simulink model "IdentificareBuclaExterna"  (R2023b)
settings: Solver=FixedStepAuto  StartTime=0.0  StopTime=2500  FixedStep=0.01  RelTol=1e-3
values from neighbouring files (symbols this model uses):
  A = 332.5    [CodDatepersonale.m]    (also in CodProiect.m; untitled.m; untitled2.m = [O I; O O]; untitled22.m)
  C = 7.4    [CodDatepersonale.m]    (also in CodProiect.m = 9; untitled.m; untitled22.m = 9)
  k = 0.036    [CodDatepersonale.m]    (also in CodProiect.m = 0.035; untitled.m; untitled22.m = 0.035)
  k1 = 0.624    [CodDatepersonale.m]    (also in CodProiect.m = 0.654; untitled.m = 0.654; untitled22.m)
  k2 = -0.015    [CodDatepersonale.m]    (also in CodProiect.m; untitled.m; untitled22.m)
  k3 = -0.0006    [CodDatepersonale.m]    (also in CodProiect.m; untitled.m; untitled22.m)
  keta = 8*10^(-5)    (= 8e-05)    [CodDatepersonale.m]    (also in CodProiect.m; untitled.m; untitled22.m)
libraries: slpidlib x1
settings Model: Creator=Daniela  LastModifiedBy=Daniela

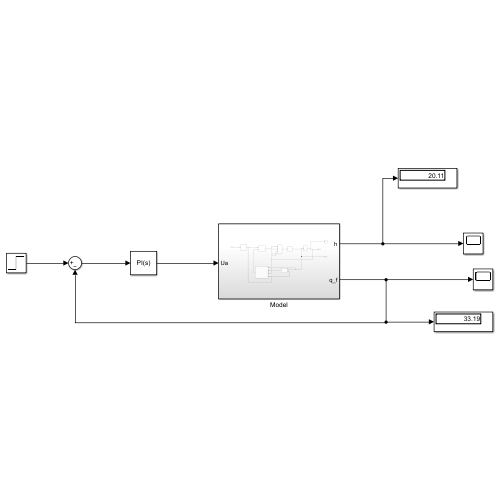
[thumbnail: Simulink's stored preview of the top-level diagram]
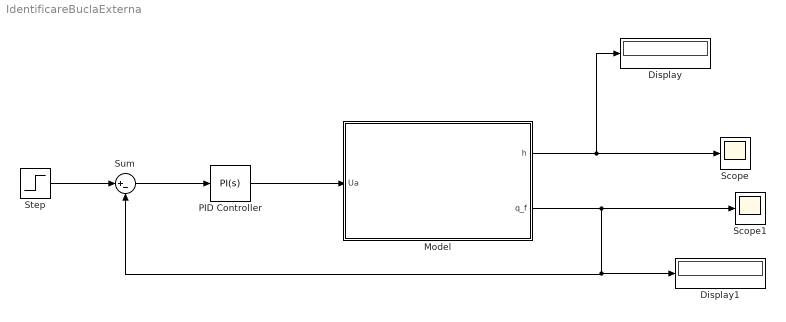
== system IdentificareBuclaExterna ==
  Display : Display
  Display1 : Display
  Model : Subsystem
  PID Controller : slpidlib/PID Controller  Controller=PI  Form=Parallel  TimeDomain=Continuous-time  UseExternalTs=off  SampleTime=-1  IntegratorMethod=Forward Euler  FilterMethod=Forward Euler  ControllerParametersSource=internal  P=0.0698  I=0.0698*1/0.784  UseKiTs=off  D=0  N=100  UseFilter=on  TunerSelectOption=Transfer Function Based (PID Tuner App)  InitialConditionSource=internal  InitialConditionForIntegrator=5.6  InitialConditionForFilter=0  DifferentiatorICPrevScaledInput=0  ExternalReset=none  TrackingMode=off  Kt=1  LimitOutput=off  SatLimitsSource=internal  UpperSaturationLimit=inf  LowerSaturationLimit=-inf  LinearizeAsGain=on  AntiWindupMode=none  Kb=1  LimitIntegrator=off  UpperIntegratorSaturationLimit=inf  LowerIntegratorSaturationLimit=-inf  POutMin=[]  POutMax=[]  IOutMin=[]  IOutMax=[]  DOutMin=[]  DOutMax=[]  NOutMin=[]  NOutMax=[]  SumOutMin=[]  SumOutMax=[]  SaturationOutMin=[]  SaturationOutMax=[]  PParamMin=[]  PParamMax=[]  IParamMin=[]  IParamMax=[]  DParamMin=[]  DParamMax=[]  NParamMin=[]  NParamMax=[]  KbParamMin=[]  KbParamMax=[]  KtParamMin=[]  KtParamMax=[]  KbOutMin=[]  KbOutMax=[]  KtOutMin=[]  KtOutMax=[]  IntegratorOutMin=[]  IntegratorOutMax=[]  FilterOutMin=[]  FilterOutMax=[]  SumI1OutMin=[]  SumI1OutMax=[]  SumI2OutMin=[]  SumI2OutMax=[]  SumI3OutMin=[]  SumI3OutMax=[]  SumI4OutMin=[]  SumI4OutMax=[]  SumDOutMin=[]  SumDOutMax=[]  DifferentiatorOutMin=[]  DifferentiatorOutMax=[]  FilterDiffOutCoefMin=[]  FilterDiffOutCoefMax=[]  ReciprocalOutMin=[]  ReciprocalOutMax=[]  SumDenOutMin=[]  SumDenOutMax=[]  SumNumOutMin=[]  SumNumOutMax=[]  DivideOutMin=[]  DivideOutMax=[]  UdiffTsProdOutMin=[]  UdiffTsProdOutMax=[]  NTsProdOutMin=[]  NTsProdOutMax=[]  UintegralTsProdOutMin=[]  UintegralTsProdOutMax=[]  UngainTsProdOutMin=[]  UngainTsProdOutMax=[]  ClampingZeroOutDataTypeStr=Inherit: Inherit via back propagation  ClampingZeroOutMin=[]  ClampingZeroOutMax=[]  FilterDenConstantOutDataTypeStr=Inherit: Inherit via back propagation  FilterDenConstantOutMin=[]  FilterDenConstantOutMax=[]  PCopyOutDataTypeStr=Inherit: Inherit via back propagation  PCopyOutMin=[]  PCopyOutMax=[]  NCopyOutDataTypeStr=Inherit: Inherit via back propagation  NCopyOutMin=[]  NCopyOutMax=[]  IntegratorContinuousStateAttributes=''  IntegratorStateMustResolveToSignalObject=off  IntegratorRTWStateStorageClass=Auto  FilterContinuousStateAttributes=''  FilterStateMustResolveToSignalObject=off  FilterRTWStateStorageClass=Auto  ParallelPVariant=InternalParameters  IdealPVariant=Disabled  IVariant=InternalParameters  DVariant=Disabled  IntegratorVariant=Continuous  SatVariant=Disabled  AWVariant=Passthrough  PCopyVariant=Disabled  TRVariant=Disabled  FdbkBlocksVariant=Forward  IdealPFdbkVariant=Disabled  SatFdbkVariant=Disabled  DerivativeFilterVariant=Disabled  NVariant=Disabled  NCopyVariant=Disabled_SignalSpec  FilterICVariant=Disabled  IntegratorICVariant=InternalICs  ExternalResetVariant=Disabled  TRSumVariant=Passthrough  SumFdbkVariant=Disabled  SumVariant=Sum_PI  TsampFilterVariant=InternalTs  TsampNgainVariant=Passthrough  TsampIntegralVariant=Disabled_SignalSpec  ExternalSaturationOutDataTypeStr=Inherit: Same as second input
  Scope : Scope
  Scope1 : Scope
  Step : Step  Time=0  Before=30.22  After=33.19  SampleTime=0
  Sum : Sum  Inputs=|+-
  wires:
  PID Controller/1 -> Model/1(Ua)
  Model/1(h) -> Display/1, Scope/1
  Model/2(q_f) -> Sum/2, Display1/1, Scope1/1
  Sum/1 -> PID Controller/1
  Step/1 -> Sum/1

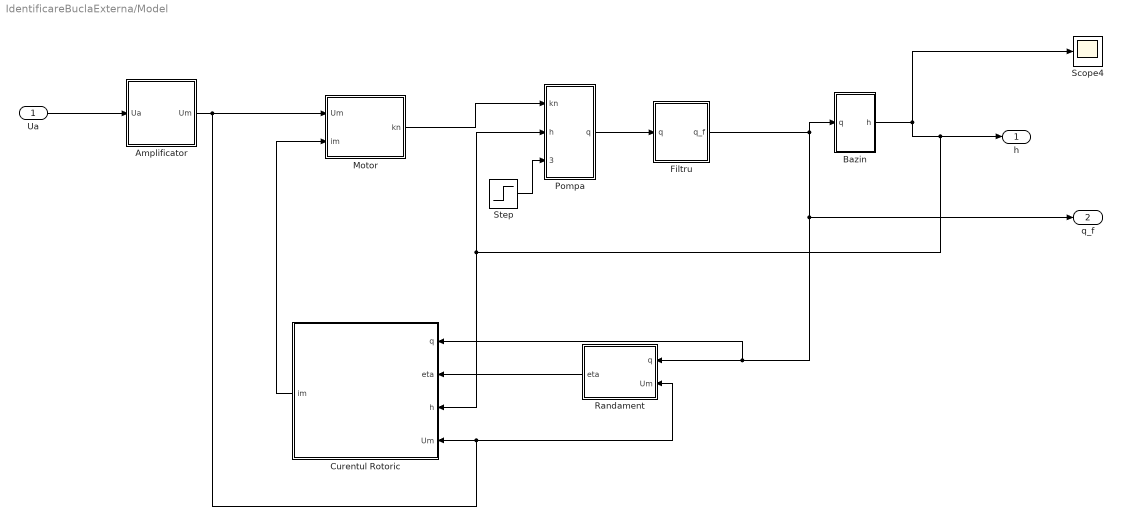
== system IdentificareBuclaExterna/Model ==
  Ua : Inport
  Amplificator : Subsystem
  Bazin : Subsystem
  Curentul Rotoric : Subsystem
  Filtru : Subsystem
  Motor : Subsystem
  Pompa : Subsystem
  Randament : Subsystem
  Scope4 : Scope
  Step : Step  Time=250  After=0.0036  SampleTime=0
  h : Outport
  q_f : Outport  Port=2
  wires:
  Bazin/1(h) -> Scope4/1, h/1, Pompa/2(h), Curentul Rotoric/3(h)
  Randament/1(eta) -> Curentul Rotoric/2(eta)
  Pompa/1(q) -> Filtru/1(q)
  Ua/1 -> Amplificator/1(Ua)
  Step/1 -> Pompa/3(Perturbatie k)
  Motor/1(kn) -> Pompa/1(kn)
  Filtru/1(q_f) -> q_f/1, Randament/1(q), Curentul Rotoric/1(q), Bazin/1(q)
  Curentul Rotoric/1(im) -> Motor/2(im)
  Amplificator/1(Um) -> Motor/1(Um), Randament/2(Um), Curentul Rotoric/4(Um)

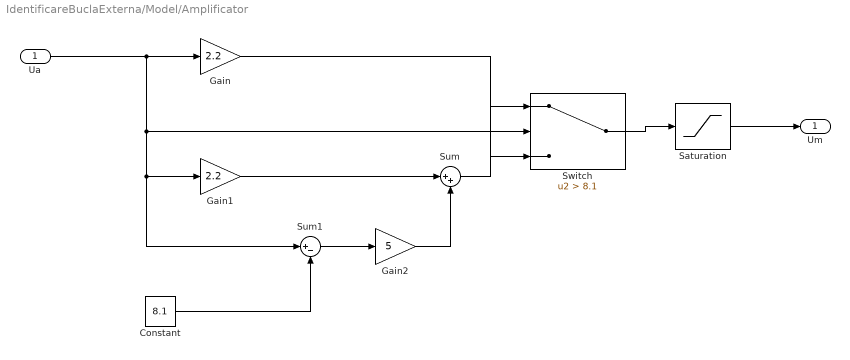
== system IdentificareBuclaExterna/Model/Amplificator ==
  Ua : Inport
  Constant : Constant  Value=8.1
  Gain : Gain  Gain=2.2
  Gain1 : Gain  Gain=2.2
  Gain2 : Gain  Gain=5
  Saturation : Saturate  UpperLimit=22  LowerLimit=0  ZeroCross=off
  Sum : Sum  Inputs=|++
  Sum1 : Sum  Inputs=|+-
  Switch : Switch  Criteria=u2 > Threshold  Threshold=8.1  SaturateOnIntegerOverflow=off  InputSameDT=off
  Um : Outport
  wires:
  Switch/1 -> Saturation/1
  Ua/1 -> Sum1/1, Gain1/1, Switch/2, Gain/1
  Constant/1 -> Sum1/2
  Sum1/1 -> Gain2/1
  Gain/1 -> Switch/3
  Sum/1 -> Switch/1
  Gain1/1 -> Sum/1
  Gain2/1 -> Sum/2
  Saturation/1 -> Um/1

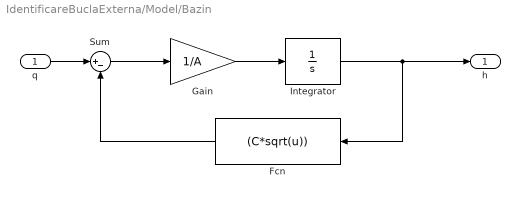
== system IdentificareBuclaExterna/Model/Bazin ==
  q : Inport
  Fcn : Fcn  Expr=(C*sqrt(u))
  Gain : Gain  Gain=1/A
  Integrator : Integrator  InitialCondition=16.53
  Sum : Sum  Inputs=|+-
  h : Outport
  wires:
  q/1 -> Sum/1
  Sum/1 -> Gain/1
  Fcn/1 -> Sum/2
  Gain/1 -> Integrator/1
  Integrator/1 -> h/1, Fcn/1

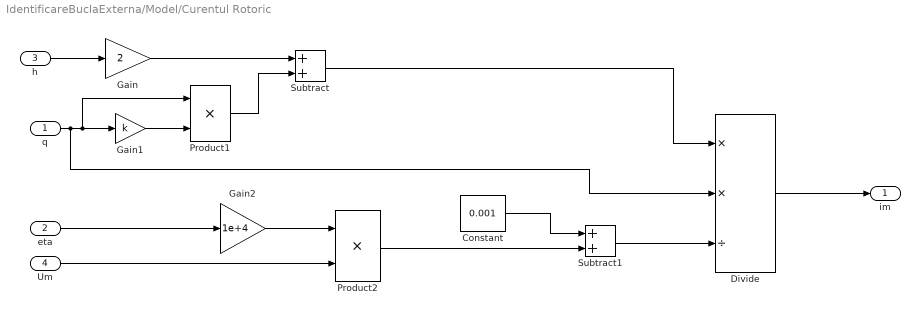
== system IdentificareBuclaExterna/Model/Curentul Rotoric ==
  q : Inport
  eta : Inport  Port=2
  h : Inport  Port=3
  Um : Inport  Port=4
  Constant : Constant  Value=0.001
  Divide : Product  Inputs=**/
  Gain : Gain  Gain=2
  Gain1 : Gain  Gain=k
  Gain2 : Gain  Gain=1e+4
  Product1 : Product
  Product2 : Product
  Subtract : Sum
  Subtract1 : Sum
  im : Outport
  wires:
  Product1/1 -> Subtract/2
  Um/1 -> Product2/2
  q/1 -> Gain1/1, Product1/1, Divide/2
  Subtract/1 -> Divide/1
  Divide/1 -> im/1
  Subtract1/1 -> Divide/3
  Gain2/1 -> Product2/1
  h/1 -> Gain/1
  Gain/1 -> Subtract/1
  Gain1/1 -> Product1/2
  eta/1 -> Gain2/1
  Product2/1 -> Subtract1/2
  Constant/1 -> Subtract1/1

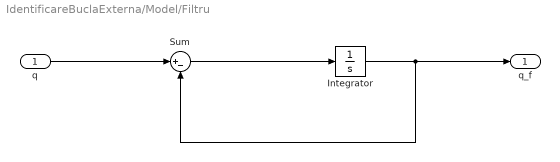
== system IdentificareBuclaExterna/Model/Filtru ==
  q : Inport
  Integrator : Integrator  InitialCondition=30.22
  Sum : Sum  Inputs=|+-
  q_f : Outport
  wires:
  Integrator/1 -> q_f/1, Sum/2
  q/1 -> Sum/1
  Sum/1 -> Integrator/1

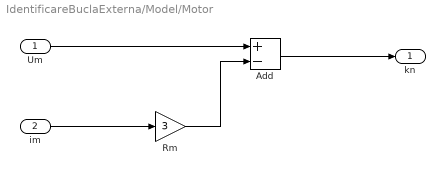
== system IdentificareBuclaExterna/Model/Motor ==
  Um : Inport
  im : Inport  Port=2
  Add : Sum  Inputs=+-
  Rm : Gain  Gain=3
  kn : Outport
  wires:
  im/1 -> Rm/1
  Add/1 -> kn/1
  Um/1 -> Add/1
  Rm/1 -> Add/2

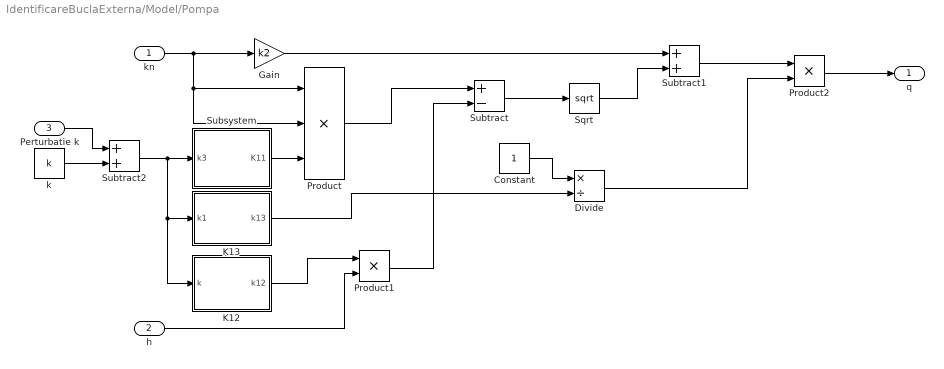
== system IdentificareBuclaExterna/Model/Pompa ==
  kn : Inport
  h : Inport  Port=2
  Perturbatie k : Inport  Port=3
  Constant : Constant
  Divide : Product  Inputs=*/
  Gain : Gain  Gain=k2
  K12 : Subsystem
  K13 : Subsystem
  Product : Product  Inputs=3
  Product1 : Product
  Product2 : Product
  Sqrt : Sqrt
  Subsystem : Subsystem
  Subtract : Sum  Inputs=+-
  Subtract1 : Sum
  Subtract2 : Sum
  k : Constant  Value=k
  q : Outport
  wires:
  K12/1(k12) -> Product1/1
  Product2/1 -> q/1
  Subtract1/1 -> Product2/1
  Product/1 -> Subtract/1
  Subtract/1 -> Sqrt/1
  Divide/1 -> Product2/2
  Product1/1 -> Subtract/2
  Subtract2/1 -> Subsystem/1(k3), K12/1(k), K13/1(k1)
  k/1 -> Subtract2/2
  K13/1(k13) -> Divide/2
  Perturbatie k/1 -> Subtract2/1
  Gain/1 -> Subtract1/1
  Subsystem/1(K11) -> Product/3
  Constant/1 -> Divide/1
  h/1 -> Product1/2
  Sqrt/1 -> Subtract1/2
  kn/1 -> Product/2, Product/1, Gain/1

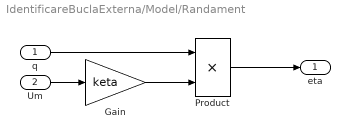
== system IdentificareBuclaExterna/Model/Randament ==
  q : Inport
  Um : Inport  Port=2
  Gain : Gain  Gain=keta
  Product : Product
  eta : Outport
  wires:
  Gain/1 -> Product/2
  Product/1 -> eta/1
  Um/1 -> Gain/1
  q/1 -> Product/1

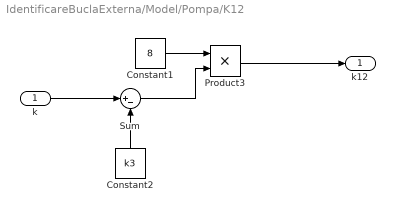
== system IdentificareBuclaExterna/Model/Pompa/K12 ==
  k : Inport
  Constant1 : Constant  Value=8
  Constant2 : Constant  Value=k3
  Product3 : Product
  Sum : Sum  Inputs=|+-
  k12 : Outport
  wires:
  Sum/1 -> Product3/2
  k/1 -> Sum/1
  Constant1/1 -> Product3/1
  Product3/1 -> k12/1
  Constant2/1 -> Sum/2

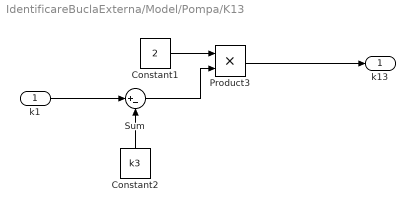
== system IdentificareBuclaExterna/Model/Pompa/K13 ==
  k1 : Inport
  Constant1 : Constant  Value=2
  Constant2 : Constant  Value=k3
  Product3 : Product
  Sum : Sum  Inputs=|+-
  k13 : Outport
  wires:
  Constant1/1 -> Product3/1
  Product3/1 -> k13/1
  Constant2/1 -> Sum/2
  k1/1 -> Sum/1
  Sum/1 -> Product3/2

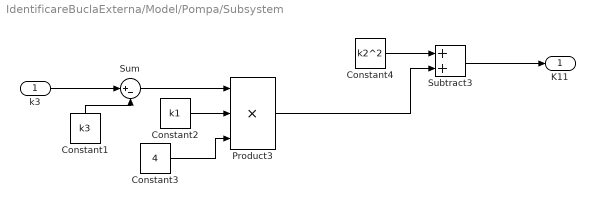
== system IdentificareBuclaExterna/Model/Pompa/Subsystem ==
  k3 : Inport
  Constant1 : Constant  Value=k3
  Constant2 : Constant  Value=k1
  Constant3 : Constant  Value=4
  Constant4 : Constant  Value=k2^2
  Product3 : Product  Inputs=3
  Subtract3 : Sum
  Sum : Sum  Inputs=|+-
  K11 : Outport
  wires:
  k3/1 -> Sum/1
  Subtract3/1 -> K11/1
  Product3/1 -> Subtract3/2
  Constant4/1 -> Subtract3/1
  Sum/1 -> Product3/1
  Constant1/1 -> Sum/2
  Constant3/1 -> Product3/3
  Constant2/1 -> Product3/2
